simulink model "spec_avg_CRD"  (R2025b)
settings: Solver=FixedStepDiscrete  StartTime=0.0  StopTime=0.0005  FixedStep=1/Fs  RelTol=1e-3
undefined symbols (not defined in the file): Add, chirp_counts, chirp_outputs, FFT_LENGTH, Fs, h, N, Shift, specAvg, T, Ts
libraries: hdlsllib x3, dsphdlsigops2 x2, dsphdlxfrm2 x1, dsphdlmathfun2 x1
settings Model: MinMaxOverflowLogging=MinMaxAndOverflow  FPTRunName=BaselineRun  FPTShortcutValueString='{{},{''BaselineRun'',1,1,1,''BaselineRun'','''',{},''M'','''',''''},{''EmbeddedRun'',1,1,1,''EmbeddedRun'','''',{},''M'','''',''''},{''BaselineRun_2'',1,1,1,''BaselineRun_2'','''',{},''M'','''',''''},{''BaselineRun_3'',1,1,1,''BaselineRun_3'','''',{},''M'','''',''''},{''BaselineRun_4'',1,1,1,''BaselineRun_4'','''',{},''M'','''',''''},{''BaselineRun_5'',1,1,1,''BaselineRun_5'','''',{},''M'','''',''''}}'  Creator=caleb  LastModifiedBy=caleb
settings OptimizationCC: BlockReduction=off  ConditionallyExecuteInputs=off  DefaultParameterBehavior=Inlined  OptimizeBlockIOStorage=off  EnhancedBackFolding=on  PassReuseOutputArgsThreshold=0.0  OptimizeBlockOrder=speed  DifferentSizesBufferReuse=on
settings DebuggingCC: SignalRangeChecking=warning  AlgebraicLoopMsg=error  SingleTaskRateTransMsg=error  ParameterTunabilityLossMsg=error
settings HardwareCC: ProdBitPerPointer=32.0  ProdBitPerSizeT=32.0  ProdBitPerPtrDiffT=32.0  ProdLargestAtomicFloat=None  ProdIntDivRoundTo=Undefined  ProdEndianess=Unspecified  ProdWordSize=32.0  ProdHWDeviceType=ASIC/FPGA->ASIC/FPGA  TargetBitPerPointer=64.0  TargetBitPerSizeT=64.0  TargetBitPerPtrDiffT=64.0  TargetLongLongMode=on  TargetIntDivRoundTo=Zero  TargetEndianess=LittleEndian  TargetWordSize=64.0  TargetHWDeviceType=Generic->Custom  ProdEqTarget=off
settings SFSimCC: MATLABDynamicMemAlloc=off
settings RTWCC: GPUComputeCapability=3.5
settings CodeAppCC: ForceParamTrailComments=on  MaxIdLength=256.0  OperatorAnnotations=on

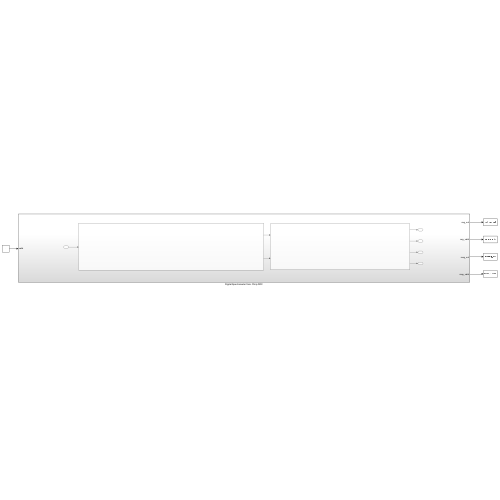
[thumbnail: Simulink's stored preview of the top-level diagram]
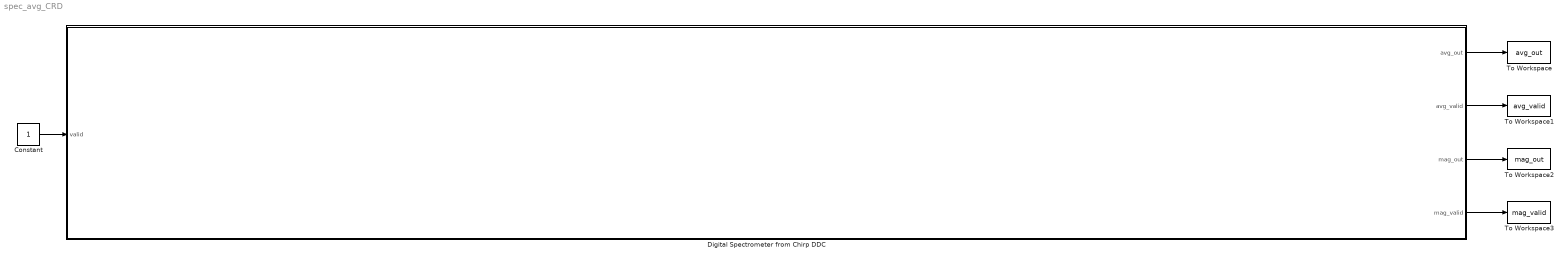
== system spec_avg_CRD ==
  Constant : Constant  OutDataTypeStr=boolean  SampleTime=1/Fs
  Digital Spectrometer from Chirp DDC : Subsystem
  To Workspace : ToWorkspace  VariableName=avg_out  SampleTime=-1
      settings: Save2DSignal=2-D array (concatenate along first dimension)
  To Workspace1 : ToWorkspace  VariableName=avg_valid  SampleTime=-1
      settings: Save2DSignal=2-D array (concatenate along first dimension)
  To Workspace2 : ToWorkspace  VariableName=mag_out  SampleTime=-1
      settings: Save2DSignal=2-D array (concatenate along first dimension)
  To Workspace3 : ToWorkspace  VariableName=mag_valid  SampleTime=-1
      settings: Save2DSignal=2-D array (concatenate along first dimension)
  wires:
  Digital Spectrometer from Chirp DDC/3(mag_out) -> To Workspace2/1
  Digital Spectrometer from Chirp DDC/1(avg_out) -> To Workspace/1
  Constant/1 -> Digital Spectrometer from Chirp DDC/1(valid)
  Digital Spectrometer from Chirp DDC/2(avg_valid) -> To Workspace1/1
  Digital Spectrometer from Chirp DDC/4(mag_valid) -> To Workspace3/1

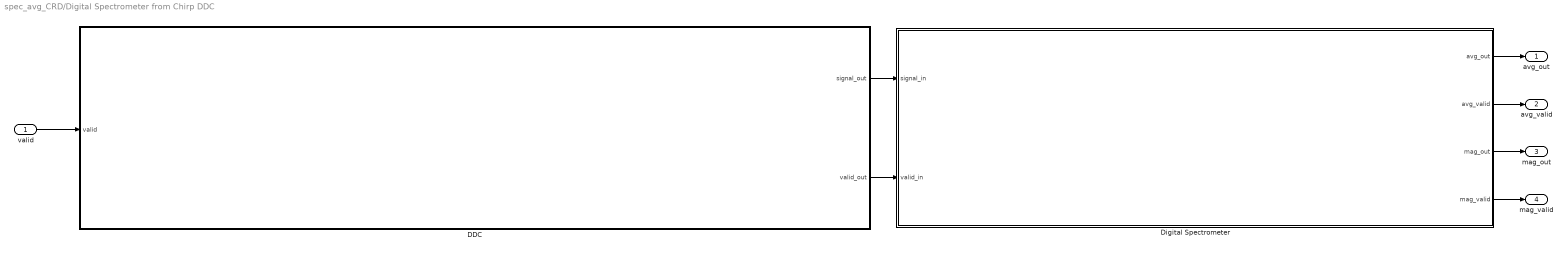
== system spec_avg_CRD/Digital Spectrometer from Chirp DDC ==
  valid : Inport
  DDC : Subsystem
  Digital Spectrometer : Subsystem
  avg_out : Outport
  avg_valid : Outport  Port=2
  mag_out : Outport  Port=3
  mag_valid : Outport  Port=4
  wires:
  Digital Spectrometer/2(avg_valid) -> avg_valid/1
  DDC/2(valid_out) -> Digital Spectrometer/2(valid_in)
  Digital Spectrometer/1(avg_out) -> avg_out/1
  valid/1 -> DDC/1(valid)
  DDC/1(signal_out) -> Digital Spectrometer/1(signal_in)
  Digital Spectrometer/4(mag_valid) -> mag_valid/1
  Digital Spectrometer/3(mag_out) -> mag_out/1

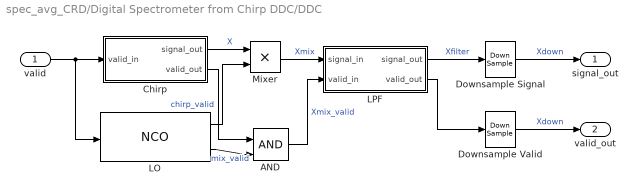
== system spec_avg_CRD/Digital Spectrometer from Chirp DDC/DDC ==
  valid : Inport
  AND : Logic  IconShape=distinctive  AllPortsSameDT=off  OutDataTypeStr=boolean
  Chirp : Subsystem
  Downsample Signal : DownSample  RateOptions=Allow multirate processing
  Downsample Valid : DownSample  RateOptions=Allow multirate processing
  LO : dsphdlsigops2/NCO  PhaseIncrementSource=Property  PhaseIncrement=phIncr  PhaseOffsetSource=Property  PhaseOffset=phOff  DitherSource=Property  NumDitherBits=ditherBits  SamplesPerFrame=1  LUTCompress=off  ResetAction=off  Waveform=Cosine  PhasePort=off  SimulateUsing=Code generation  AccumulatorWL=N  PhaseQuantization=on  NumQuantizerAccumulatorBits=Q  OutputDataType=Binary point scaling  OutputWL=16  OutputFL=14
  LPF : Subsystem
  Mixer : Product  OutDataTypeStr=fixdt(1,16,14)
  signal_out : Outport  VectorParamsAs1DForOutWhenUnconnected=off
  valid_out : Outport  Port=2  VectorParamsAs1DForOutWhenUnconnected=off
  wires:
  valid/1 -> LO/1, Chirp/1(valid_in)
  LPF/1(signal_out) -> Downsample Signal/1  "Xfilter"
  Chirp/1(signal_out) -> Mixer/1  "X"
  Downsample Valid/1 -> valid_out/1  "Xdown"
  Chirp/2(valid_out) -> AND/1  "chirp_valid"
  LO/1 -> Mixer/2
  Mixer/1 -> LPF/1(signal_in)  "Xmix"
  LO/2 -> AND/2  "mix_valid"
  AND/1 -> LPF/2(valid_in)  "Xmix_valid"
  LPF/2(valid_out) -> Downsample Valid/1
  Downsample Signal/1 -> signal_out/1  "Xdown"

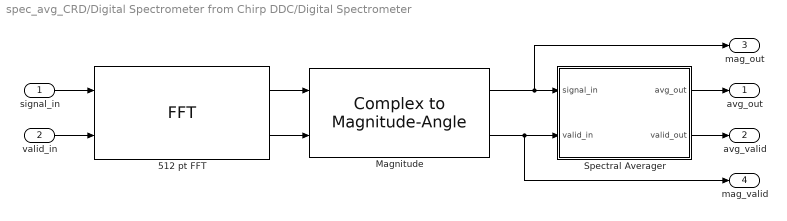
== system spec_avg_CRD/Digital Spectrometer from Chirp DDC/Digital Spectrometer ==
  signal_in : Inport
  valid_in : Inport  Port=2
  512 pt FFT : dsphdlxfrm2/FFT  Architecture=Streaming Radix 2^2  FFTLengthSource=Property  FFTLength=FFT_LENGTH  FFTLengthMax=1024  ComplexMultiplication=Use 4 multipliers and 2 adders  BitReversedOutput=off  BitReversedInput=off  Normalize=off  SimulateUsing=Code generation  RoundingMethod=Floor  ResetInputPort=off  StartOutputPort=off  EndOutputPort=off
  Magnitude : dsphdlmathfun2/Complex to Magnitude-Angle  NumIterationsSource=Auto  NumIterations=10  OutputFormat=Magnitude  AngleFormat=Normalized  ScaleOutput=off  ScalingMethod=Shift-Add  SimulateUsing=Code generation
  Spectral Averager : Subsystem
  avg_out : Outport
  avg_valid : Outport  Port=2
  mag_out : Outport  Port=3
  mag_valid : Outport  Port=4
  wires:
  Magnitude/2 -> Spectral Averager/2(valid_in), mag_valid/1
  signal_in/1 -> 512 pt FFT/1
  valid_in/1 -> 512 pt FFT/2
  512 pt FFT/1 -> Magnitude/1
  512 pt FFT/2 -> Magnitude/2
  Magnitude/1 -> Spectral Averager/1(signal_in), mag_out/1
  Spectral Averager/1(avg_out) -> avg_out/1
  Spectral Averager/2(valid_out) -> avg_valid/1

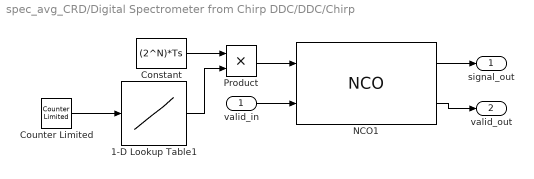
== system spec_avg_CRD/Digital Spectrometer from Chirp DDC/DDC/Chirp ==
  valid_in : Inport
  1-D Lookup Table1 : Lookup_n-D  NumberOfTableDimensions=1  LookupTableObject=''  BreakpointsForDimension1=chirp_counts  BreakpointsForDimension1FirstPoint=10  BreakpointsForDimension2FirstPoint=10  BreakpointsForDimension1Spacing=12  BreakpointsForDimension2Spacing=12  BreakpointsForDimension1DataTypeStr=uint16  IndexSearchMethod=Evenly spaced points  Table=chirp_outputs  TableDataTypeStr=uint32  InterpMethod=Flat  DiagnosticForOutOfRangeInput=Error  InternalRulePriority=Speed  OutDataTypeStr=uint32  RndMeth=Simplest  LockScale=on
  Constant : Constant  Value=(2^N)*Ts  OutDataTypeStr=fixdt(0,16,10)  SampleTime=1/Fs
  Counter Limited : hdlsllib/Sources/Counter Limited  uplimit=T/Ts  tsamp=1/Fs
  NCO1 : dsphdlsigops2/NCO  PhaseIncrementSource=Input port  PhaseIncrement=phIncr  PhaseOffsetSource=Property  PhaseOffset=phOff  DitherSource=Property  NumDitherBits=ditherBits  SamplesPerFrame=1  LUTCompress=off  ResetAction=off  Waveform=Cosine  PhasePort=off  SimulateUsing=Code generation  AccumulatorWL=N  PhaseQuantization=on  NumQuantizerAccumulatorBits=Q  OutputDataType=Binary point scaling  OutputWL=16  OutputFL=14
  Product : Product  OutDataTypeStr=uint32  LockScale=on
  signal_out : Outport
  valid_out : Outport  Port=2
  wires:
  Constant/1 -> Product/1
  Counter Limited/1 -> 1-D Lookup Table1/1
  valid_in/1 -> NCO1/2
  1-D Lookup Table1/1 -> Product/2
  Product/1 -> NCO1/1
  NCO1/1 -> signal_out/1
  NCO1/2 -> valid_out/1

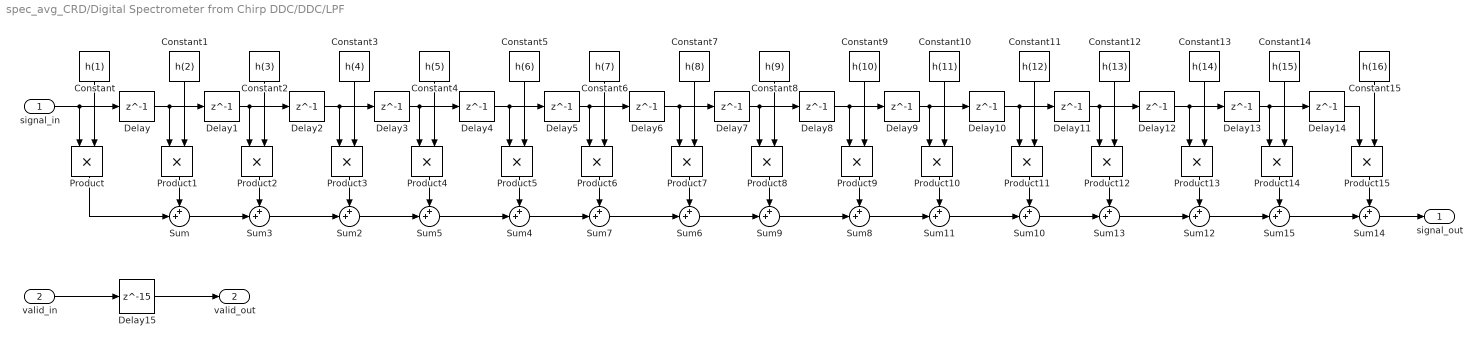
== system spec_avg_CRD/Digital Spectrometer from Chirp DDC/DDC/LPF ==
  signal_in : Inport  OutDataTypeStr=fixdt(1,16,14)
  valid_in : Inport  Port=2  OutDataTypeStr=boolean
  Constant : Constant  Value=h(1)  OutDataTypeStr=fixdt(1,16,4)  SampleTime=1/Fs
  Constant1 : Constant  Value=h(2)  OutDataTypeStr=fixdt(1,16,25)  SampleTime=1/Fs
  Constant10 : Constant  Value=h(11)  OutDataTypeStr=fixdt(0,16,19)  SampleTime=1/Fs
  Constant11 : Constant  Value=h(12)  OutDataTypeStr=fixdt(0,16,23)  SampleTime=1/Fs
  Constant12 : Constant  Value=h(13)  OutDataTypeStr=fixdt(1,16,21)  SampleTime=1/Fs
  Constant13 : Constant  Value=h(14)  OutDataTypeStr=fixdt(1,16,22)  SampleTime=1/Fs
  Constant14 : Constant  Value=h(15)  OutDataTypeStr=fixdt(1,16,25)  SampleTime=1/Fs
  Constant15 : Constant  Value=h(16)  OutDataTypeStr=fixdt(1,16,4)  SampleTime=1/Fs
  Constant2 : Constant  Value=h(3)  OutDataTypeStr=fixdt(1,16,22)  SampleTime=1/Fs
  Constant3 : Constant  Value=h(4)  OutDataTypeStr=fixdt(1,16,21)  SampleTime=1/Fs
  Constant4 : Constant  Value=h(5)  OutDataTypeStr=fixdt(0,16,23)  SampleTime=1/Fs
  Constant5 : Constant  Value=h(6)  OutDataTypeStr=fixdt(0,16,19)  SampleTime=1/Fs
  Constant6 : Constant  Value=h(7)  OutDataTypeStr=fixdt(0,16,18)  SampleTime=1/Fs
  Constant7 : Constant  Value=h(8)  OutDataTypeStr=fixdt(0,16,17)  SampleTime=1/Fs
  Constant8 : Constant  Value=h(9)  OutDataTypeStr=fixdt(0,16,17)  SampleTime=1/Fs
  Constant9 : Constant  Value=h(10)  OutDataTypeStr=fixdt(0,16,18)  SampleTime=1/Fs
  Delay{,1..14} (15 alike) : Delay  DelayLength=1  InitialCondition=0  UseCircularBuffer=on
  Delay15 : Delay  DelayLength=15
  Product : Product  OutDataTypeStr=fixdt(1,16,4)
  Product1 : Product  OutDataTypeStr=fixdt(1,16,25)
  Product10 : Product  OutDataTypeStr=fixdt(1,16,18)
  Product{2,4,11,13} (4 alike) : Product  OutDataTypeStr=fixdt(1,16,22)
  Product12 : Product  OutDataTypeStr=fixdt(1,16,21)
  Product14 : Product  OutDataTypeStr=fixdt(1,16,25)
  Product15 : Product  OutDataTypeStr=fixdt(1,16,4)
  Product3 : Product  OutDataTypeStr=fixdt(1,16,21)
  Product5 : Product  OutDataTypeStr=fixdt(1,16,18)
  Product6 : Product  OutDataTypeStr=fixdt(1,16,17)
  Product7 : Product  OutDataTypeStr=fixdt(1,16,16)
  Product8 : Product  OutDataTypeStr=fixdt(1,16,16)
  Product9 : Product  OutDataTypeStr=fixdt(1,16,17)
  Sum : Sum  Inputs=++|  OutDataTypeStr=fixdt(1,16,25)
  Sum{8,10..15} (7 alike) : Sum  Inputs=++|  OutDataTypeStr=fixdt(1,16,15)
  Sum2 : Sum  Inputs=++|  OutDataTypeStr=fixdt(1,16,21)
  Sum3 : Sum  Inputs=++|  OutDataTypeStr=fixdt(1,16,22)
  Sum4 : Sum  Inputs=++|  OutDataTypeStr=fixdt(1,16,18)
  Sum5 : Sum  Inputs=++|  OutDataTypeStr=fixdt(1,16,21)
  Sum6 : Sum  Inputs=++|  OutDataTypeStr=fixdt(1,16,16)
  Sum7 : Sum  Inputs=++|  OutDataTypeStr=fixdt(1,16,17)
  Sum9 : Sum  Inputs=++|  OutDataTypeStr=fixdt(1,16,16)
  signal_out : Outport
  valid_out : Outport  Port=2  VectorParamsAs1DForOutWhenUnconnected=off
  wires:
  signal_in/1 -> Delay/1, Product/1
  Delay/1 -> Product1/1, Delay1/1
  Constant/1 -> Product/2
  Constant1/1 -> Product1/2
  Product1/1 -> Sum/1
  Product/1 -> Sum/2
  Constant2/1 -> Product2/2
  Delay1/1 -> Delay2/1, Product2/1
  Product2/1 -> Sum3/1
  Delay2/1 -> Product3/1, Delay3/1
  Sum3/1 -> Sum2/2
  Constant3/1 -> Product3/2
  Product3/1 -> Sum2/1
  Constant4/1 -> Product4/2
  Delay3/1 -> Delay4/1, Product4/1
  Product4/1 -> Sum5/1
  Delay4/1 -> Product5/1, Delay5/1
  Sum5/1 -> Sum4/2
  Constant5/1 -> Product5/2
  Product5/1 -> Sum4/1
  Constant6/1 -> Product6/2
  Delay5/1 -> Delay6/1, Product6/1
  Product6/1 -> Sum7/1
  Delay6/1 -> Product7/1, Delay7/1
  Sum7/1 -> Sum6/2
  Constant7/1 -> Product7/2
  Product7/1 -> Sum6/1
  Constant8/1 -> Product8/2
  Delay7/1 -> Delay8/1, Product8/1
  Product8/1 -> Sum9/1
  Delay8/1 -> Product9/1, Delay9/1
  Sum9/1 -> Sum8/2
  Constant9/1 -> Product9/2
  Product9/1 -> Sum8/1
  Constant10/1 -> Product10/2
  Delay9/1 -> Delay10/1, Product10/1
  Product10/1 -> Sum11/1
  Delay10/1 -> Product11/1, Delay11/1
  Sum11/1 -> Sum10/2
  Constant11/1 -> Product11/2
  Product11/1 -> Sum10/1
  Constant12/1 -> Product12/2
  Delay11/1 -> Delay12/1, Product12/1
  Product12/1 -> Sum13/1
  Delay12/1 -> Product13/1, Delay13/1
  Sum13/1 -> Sum12/2
  Constant13/1 -> Product13/2
  Product13/1 -> Sum12/1
  Constant14/1 -> Product14/2
  Delay13/1 -> Delay14/1, Product14/1
  Product14/1 -> Sum15/1
  Delay14/1 -> Product15/1
  Sum15/1 -> Sum14/2
  Constant15/1 -> Product15/2
  Product15/1 -> Sum14/1
  Sum12/1 -> Sum15/2
  Sum10/1 -> Sum13/2
  Sum8/1 -> Sum11/2
  Sum6/1 -> Sum9/2
  Sum4/1 -> Sum7/2
  Sum2/1 -> Sum5/2
  Sum/1 -> Sum3/2
  Sum14/1 -> signal_out/1
  valid_in/1 -> Delay15/1
  Delay15/1 -> valid_out/1

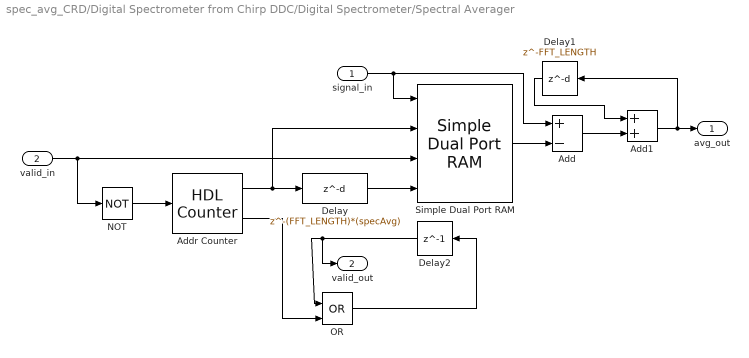
== system spec_avg_CRD/Digital Spectrometer from Chirp DDC/Digital Spectrometer/Spectral Averager ==
  signal_in : Inport  OutDataTypeStr=fixdt(1,26,15)
  valid_in : Inport  Port=2
  Add : Sum  Inputs=+-  OutDataTypeStr=fixdt(1,16,7)
  Add1 : Sum  OutDataTypeStr=fixdt(1,32,4)  AccumDataTypeStr=fixdt(1,32,4)
  Addr Counter : hdlsllib/Sources/HDL Counter  CountType=Modulo  CountInit=0  CountStep=1  CountMax=(FFT_LENGTH * specAvg)-1  CountFromType=Initial value  CountFrom=0  CountResetPort=on  CountLoadPort=off  CountEnbPort=off  CountDirPort=off  CountHitOutputPort=on  CountDataType=Unsigned  CountWordLen=log2(FFT_LENGTH)+ceil(log2(specAvg))  CountFracLen=0  CountSampTime=2/Fs
  Delay : Delay  DelayLength=(FFT_LENGTH)*(specAvg)
  Delay1 : Delay  DelayLength=FFT_LENGTH
  Delay2 : Delay  DelayLength=1
  NOT : Logic  Operator=NOT  IconShape=distinctive  AllPortsSameDT=off  OutDataTypeStr=boolean
  OR : Logic  Operator=OR  IconShape=distinctive  AllPortsSameDT=off  OutDataTypeStr=boolean
  Simple Dual Port RAM : hdlsllib/HDL RAMs/Simple Dual Port RAM  ram_size=ceil(log2(specAvg))+log2(FFT_LENGTH)
  avg_out : Outport
  valid_out : Outport  Port=2  VectorParamsAs1DForOutWhenUnconnected=off
  wires:
  valid_in/1 -> Simple Dual Port RAM/3, NOT/1
  Delay2/1 -> OR/1, valid_out/1
  OR/1 -> Delay2/1
  NOT/1 -> Addr Counter/1
  Addr Counter/1 -> Delay/1, Simple Dual Port RAM/2
  Addr Counter/2 -> OR/2
  signal_in/1 -> Simple Dual Port RAM/1, Add/1
  Delay/1 -> Simple Dual Port RAM/4
  Simple Dual Port RAM/1 -> Add/2
  Delay1/1 -> Add1/1
  Add/1 -> Add1/2
  Add1/1 -> Delay1/1, avg_out/1
